simulink model "CoPT_ThermDem"  (R2016b)
settings: configuration reference "CodeGenConfigSet" (kept outside this file)
values from neighbouring files (symbols this model uses):
  CoPT_tClntDesMax_C = Calibration.Parameter    [init_CoPT_ThermDem.m]    (also in init_CoPT_ThermDem_SIL.m = Simulink.Parameter)
  CoPT_tClntDesMin_C = Calibration.Parameter    [init_CoPT_ThermDem.m]    (also in init_CoPT_ThermDem_SIL.m = Simulink.Parameter)
libraries: CXLib x1
settings Model: Creator=Wollf  LastModifiedBy=bianxuyin
settings ConfigSetRef: SourceLocation=Base Workspace

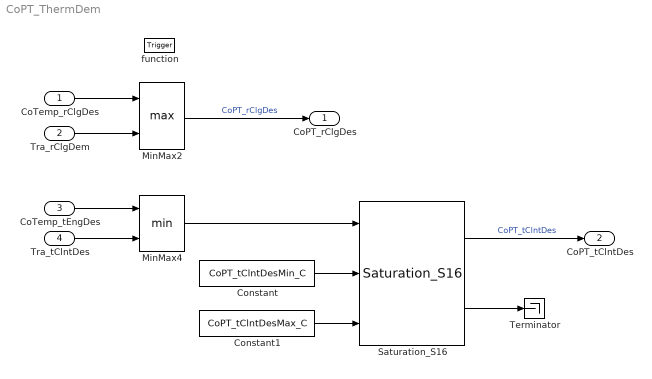
== system CoPT_ThermDem ==
  CoTemp_rClgDes : Inport  Tag=%  Description=Cooling requirement of the combustion engine  OutMin=-300  OutMax=300  OutDataTypeStr=Prc_100_rate
  Tra_rClgDem : Inport  Tag=%  Description=Relative fan cooling capacity  Port=2  OutMin=-300  OutMax=300  OutDataTypeStr=Prc_100_rate
  CoTemp_tEngDes : Inport  Tag=deg  Description=Coolant temperature of combustion engine  Port=3  OutMin=-3549  OutMax=3003  OutDataTypeStr=Temp_deg
  Tra_tClntDes : Inport  Tag=deg  Description=Coolant temperature - Set point value  Port=4  OutMin=-150  OutMax=150  OutDataTypeStr=Temp_deg
  function : TriggerPort  TriggerType=function-call  VariantControl=Variant
  Constant : Constant  Value=CoPT_tClntDesMin_C
  Constant1 : Constant  Value=CoPT_tClntDesMax_C
  MinMax2 : MinMax  Function=max  Inputs=2  InputSameDT=on
  MinMax4 : MinMax  Inputs=2  InputSameDT=on
  Saturation_S16 : CXLib/Saturation_S16
  Terminator : Terminator
  CoPT_rClgDes : Outport  Tag=%  Description=Whole cool demand of the impulse rope for the ventilator  OutMin=-300  OutMax=300  OutDataTypeStr=Prc_100_rate
  CoPT_tClntDes : Outport  Tag=deg  Description=Desired coolent temperature of the impulse rope  Port=2  OutMin=-150  OutMax=150  OutDataTypeStr=Temp_deg
  wires:
  CoTemp_tEngDes/1 -> MinMax4/1
  MinMax4/1 -> Saturation_S16/1
  MinMax2/1 -> CoPT_rClgDes/1  "CoPT_rClgDes"
  Tra_rClgDem/1 -> MinMax2/2
  CoTemp_rClgDes/1 -> MinMax2/1
  Tra_tClntDes/1 -> MinMax4/2
  Saturation_S16/1 -> CoPT_tClntDes/1  "CoPT_tClntDes"
  Constant/1 -> Saturation_S16/2
  Constant1/1 -> Saturation_S16/3
  Saturation_S16/2 -> Terminator/1
